simulink library "INT_ASMod_VolEff"  (R2016b)
settings: Solver=VariableStepAuto  StartTime=0.0  StopTime=10.0  RelTol=1e-3
settings Model: Creator=zhoukai  LastModifiedBy=zhoukai

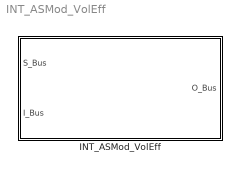
== system INT_ASMod_VolEff ==
  INT_ASMod_VolEff : Subsystem

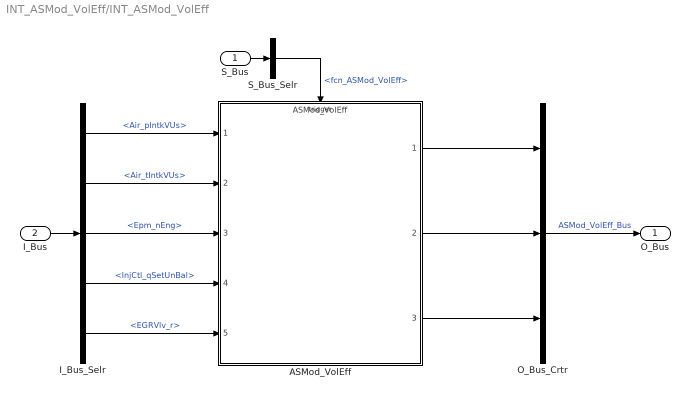
== system INT_ASMod_VolEff/INT_ASMod_VolEff ==
  S_Bus : Inport
  I_Bus : Inport  Port=2
  ASMod_VolEff : ModelReference  ModelNameDialog=ASMod_VolEff  SimulationMode=Normal  ModelReferenceVersion=1.23  TriggerPortName=function  TriggerPortTriggerType=function-call  TriggerPortStatesWhenEnabling=held
  I_Bus_Selr : BusSelector  OutputSignals=Air_pIntkVUs,Air_tIntkVUs,Epm_nEng,InjCtl_qSetUnBal,EGRVlv_r
  O_Bus_Crtr : BusCreator  Inputs=3
  S_Bus_Selr : BusSelector  OutputSignals=fcn_ASMod_VolEff
  O_Bus : Outport
  wires:
  S_Bus_Selr/1 -> ASMod_VolEff/Trigger  "<fcn_ASMod_VolEff>"
  S_Bus/1 -> S_Bus_Selr/1
  I_Bus/1 -> I_Bus_Selr/1
  I_Bus_Selr/1 -> ASMod_VolEff/1  "<Air_pIntkVUs>"
  I_Bus_Selr/2 -> ASMod_VolEff/2  "<Air_tIntkVUs>"
  I_Bus_Selr/3 -> ASMod_VolEff/3  "<Epm_nEng>"
  I_Bus_Selr/4 -> ASMod_VolEff/4  "<InjCtl_qSetUnBal>"
  I_Bus_Selr/5 -> ASMod_VolEff/5  "<EGRVlv_r>"
  O_Bus_Crtr/1 -> O_Bus/1  "ASMod_VolEff_Bus"
  ASMod_VolEff/1 -> O_Bus_Crtr/1
  ASMod_VolEff/2 -> O_Bus_Crtr/2
  ASMod_VolEff/3 -> O_Bus_Crtr/3
